simulink model "exm4_17"  (Simulink 3.00)
settings: Solver=ode45  StartTime=0.0  StopTime=1500  RelTol=1e-3

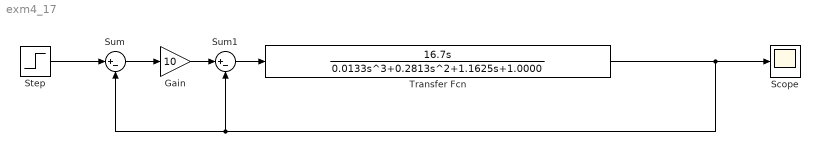
== system exm4_17 ==
  Gain : Gain  Gain=10  SaturateOnIntegerOverflow=on
  Scope : Scope
      settings: TimeRange=1500  YMin=-0.2  YMax=1.6  SaveToWorkspace=off  SaveName=ScopeData  LimitMaxRows=off
  Step : Step  Time=0  Before=0  After=1  SampleTime=0
  Sum : Sum  Inputs=|+-  SaturateOnIntegerOverflow=on
  Sum1 : Sum  Inputs=|+-  SaturateOnIntegerOverflow=on
  Transfer Fcn : TransferFcn  Numerator=[16.7 0]  Denominator="[0.0133    0.2813    1.1625    1.0000]"
  wires:
  Step/1 -> Sum/1
  Sum/1 -> Gain/1
  Gain/1 -> Sum1/1
  Sum1/1 -> Transfer Fcn/1
  Transfer Fcn/1 -> Scope/1, Sum1/2, Sum/2
